simulink model "Model_FluidFlow_14b"  (R2014b)
settings: Solver=ode45  StartTime=0.0  StopTime=800  RelTol=1e-3
undefined symbols (not defined in the file or in its folder): in, param
settings Model: Creator=Arek  LastModifiedBy=Arek
settings SolverCC: ZeroCrossAlgorithm=Adaptive

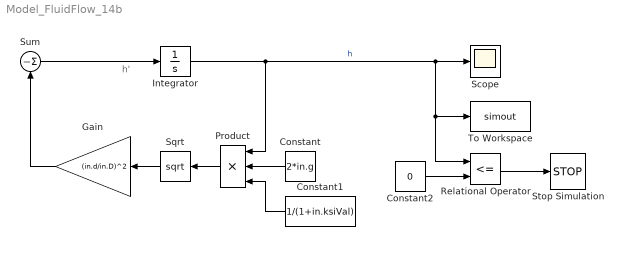
== system Model_FluidFlow_14b ==
  note: h'
  Constant : Constant  Value=2*in.g
  Constant1 : Constant  Value=1/(1+in.ksiVal)  VectorParams1D=off
  Constant2 : Constant  Value=0
  Gain : Gain  Gain=(in.d/in.D)^2
  Integrator : Integrator  InitialCondition=param.ic
  Product : Product  Inputs=3
  Relational Operator : RelationalOperator  Operator=<=  OutDataTypeStr=boolean
  Scope : Scope
      settings: TimeRange=64.93538629774619  YMin=-1
  Sqrt : Sqrt  SaturateOnIntegerOverflow=on
  Stop Simulation : Stop
  Sum : Sum  Inputs=|-
  To Workspace : ToWorkspace  VariableName=simout  SaveFormat=Timeseries  SampleTime=-1
  wires:
  Integrator/1 -> Product/1, Relational Operator/1, To Workspace/1, Scope/1  "h"
  Sum/1 -> Integrator/1
  Gain/1 -> Sum/1
  Constant/1 -> Product/2
  Constant1/1 -> Product/3
  Relational Operator/1 -> Stop Simulation/1
  Constant2/1 -> Relational Operator/2
  Product/1 -> Sqrt/1
  Sqrt/1 -> Gain/1
